simulink model "Lec_04_Storage10kWh"  (R2019b)
settings: Solver=VariableStepAuto  StartTime=0.0  StopTime=8400*3  MaxStep=0.05  RelTol=1e-3
undefined symbols (not defined in the file): Tcell0
libraries: simulink x5
settings Model: Creator=matm  LastModifiedBy=matm
settings SolverCC: ShapePreserveControl=EnableAll  SolverResetMethod=Robust
settings DataIOCC: ReturnWorkspaceOutputs=off
settings DebuggingCC: ArithmeticOperatorsInVariantConditions=warning
settings SFSimCC: SimUseLocalCustomCode=off  CustomCodeUndefinedFunction=UseInterfaceOnly
settings RTWCC: RTWUseLocalCustomCode=off
settings CodeAppCC: StateflowObjectComments=on

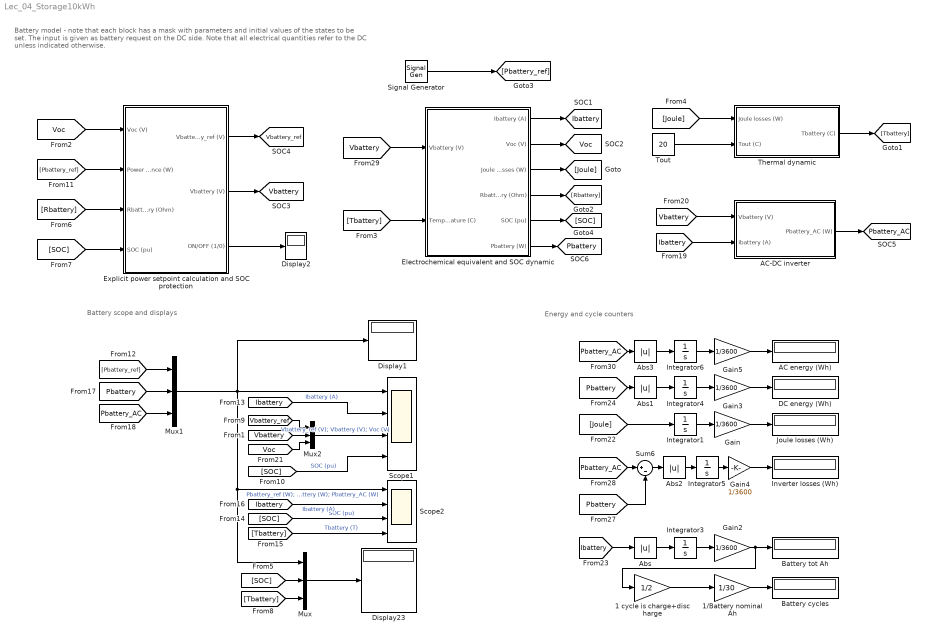
== system Lec_04_Storage10kWh ==
  note: Battery model - note that each block has a mask with parameters and initial values of the states to be set. The input is given as battery request on the DC side.
      | Note that all electrical quantities refer to the DC unless indicated otherwise.
  note: Battery scope and displays
  note: Energy and cycle counters
  1 cycle is charge+discharge : Gain  Gain=1/2
  1/Battery nominal Ah : Gain  Gain=1/30
  AC energy (Wh) : Display
  AC-DC inverter : Subsystem  mask{Inverter_Efficiency=0.95, Inverter_latency=0.1}
      mask prompts: Inverter_Efficiency "Inverter efficiency (pu)"; Inverter_latency "Inverter latency (s)"
  Abs{,1..3} (4 alike) : Abs
  Battery cycles : Display
  Battery tot Ah : Display
  DC energy (Wh) : Display
  Display1 : Display
  Display2 : Display
  Display23 : Display
  Electrochemical equivalent and SOC dynamic : Subsystem  mask{NumCellsSeries=100, NumCellsParallel=10, Ccell=3, SOC0=1}
      mask prompts: NumCellsSeries "Number of cells in Series"; NumCellsParallel "Number of cells in Parallel"; Ccell "Cell capacity (Ah)"; SOC0 "Initial state of charge (pu)"
  Explicit power setpoint calculation and SOC protection : Subsystem  mask{SOC_Max=1, SOC_Min=0, NumCellsSeries=100, CellVoltage_Max=4.2, CellVoltage_Min=2.6}
      mask prompts: SOC_Max "Max SOC (pu)"; SOC_Min "Min SOC (pu)"; NumCellsSeries "Number of celles in series"; CellVoltage_Max "Max cell voltage (V)"; CellVoltage_Min "Min cell voltage (V)"
      mask DialogControl DescTextVar Prompt: Power calculations and protections
  Gain{,2..5} (5 alike) : Gain  Gain=1/3600
  Integrator{1,3..6} (5 alike) : Integrator
  Inverter losses (Wh) : Display
  Joule losses (Wh) : Display
  Mux : Mux  Inputs=3
  Mux1 : Mux  Inputs=3
  Mux2 : Mux  Inputs=3
  Scope1 : Scope  NumInputPorts=4
  Scope2 : Scope  NumInputPorts=4
  Signal Generator : SignalGenerator  WaveForm=square  Amplitude=-10800  Frequency=1/(4200*2)
  Sum6 : Sum  Inputs=|+-
  Thermal dynamic : Subsystem  mask{Cth=72000, Rth=0.2}
      mask prompts: Cth "Thermal Capacitance (J/K)"; Rth "Thermal Resistance (K/W)"
      mask DialogControl DescTextVar Prompt: Thermal dynamic
  Tout : Constant  Value=20
  tag scope: Ibattery=global, Pbattery=global, Pbattery_AC=global, Vbattery=global, Vbattery_ref=global, Voc=global
  wires:
  [Vbattery] -> Electrochemical equivalent and SOC dynamic/1(Vbattery (V))
  Electrochemical equivalent and SOC dynamic/1(Ibattery (A)) -> [Ibattery]
  [Voc] -> Explicit power setpoint calculation and SOC protection/1(Voc (V))
  Electrochemical equivalent and SOC dynamic/2(Voc (V)) -> [Voc]
  Explicit power setpoint calculation and SOC protection/2(Vbattery (V)) -> [Vbattery]
  Electrochemical equivalent and SOC dynamic/3(Joule losses (W)) -> [Joule]
  Tout/1 -> Thermal dynamic/2(Tout (C))
  [Tbattery] -> Electrochemical equivalent and SOC dynamic/2(Temperature (C))
  Thermal dynamic/1(Tbattery (C)) -> [Tbattery]
  Mux/1 -> Display23/1
  Electrochemical equivalent and SOC dynamic/4(Rbattery (Ohm)) -> [Rbattery]
  [Rbattery] -> Explicit power setpoint calculation and SOC protection/3(Rbattery (Ohm))
  [SOC] -> Explicit power setpoint calculation and SOC protection/4(SOC (pu))
  Mux1/1 -> Display1/1, Scope1/1, Scope2/1, Mux/1  "Pbattery_ref (W); Pbattery (W); Pbattery_AC (W)"
  Explicit power setpoint calculation and SOC protection/3(ON/OFF (1/0)) -> Display2/1
  [Tbattery] -> Mux/3
  [Pbattery] -> Mux1/2
  [Pbattery_ref] -> Explicit power setpoint calculation and SOC protection/2(Power reference (W))
  [Pbattery_ref] -> Mux1/1
  [SOC] -> Scope1/4  "SOC (pu)"
  [Ibattery] -> Scope1/2  "Ibattery (A)"
  [SOC] -> Scope2/3  "SOC (pu)"
  [Tbattery] -> Scope2/4  "Tbattery (T)"
  [Ibattery] -> Scope2/2  "Ibattery (A)"
  Electrochemical equivalent and SOC dynamic/5(SOC (pu)) -> [SOC]
  Explicit power setpoint calculation and SOC protection/1(Vbattery_ref (V)) -> [Vbattery_ref]
  [Joule] -> Thermal dynamic/1(Joule losses (W))
  [Vbattery] -> AC-DC inverter/1(Vbattery (V))
  [Ibattery] -> AC-DC inverter/2(Ibattery (A))
  Electrochemical equivalent and SOC dynamic/6(Pbattery (W)) -> [Pbattery]
  [Pbattery_AC] -> Mux1/3
  [SOC] -> Mux/2
  AC-DC inverter/1(Pbattery_AC (W)) -> [Pbattery_AC]
  Mux2/1 -> Scope1/3  "Vbattery_ref (V); Vbattery (V); Voc (V)"
  [Vbattery] -> Mux2/2
  1/Battery nominal Ah/1 -> Battery cycles/1
  Integrator6/1 -> Gain5/1
  Gain2/1 -> 1 cycle is charge+discharge/1, Battery tot Ah/1
  [Pbattery_AC] -> Sum6/1
  Integrator5/1 -> Gain4/1
  [Pbattery_AC] -> Abs3/1
  Abs2/1 -> Integrator5/1
  Abs3/1 -> Integrator6/1
  Gain3/1 -> DC energy (Wh)/1
  Gain4/1 -> Inverter losses (Wh)/1
  Sum6/1 -> Abs2/1
  Integrator4/1 -> Gain3/1
  Abs1/1 -> Integrator4/1
  Integrator3/1 -> Gain2/1
  [Ibattery] -> Abs/1
  Gain/1 -> Joule losses (Wh)/1
  Integrator1/1 -> Gain/1
  Abs/1 -> Integrator3/1
  [Pbattery] -> Abs1/1
  [Joule] -> Integrator1/1
  [Pbattery] -> Sum6/2
  Gain5/1 -> AC energy (Wh)/1
  Signal Generator/1 -> [Pbattery_ref]
  [Vbattery_ref] -> Mux2/1
  [Voc] -> Mux2/3
  1 cycle is charge+discharge/1 -> 1/Battery nominal Ah/1

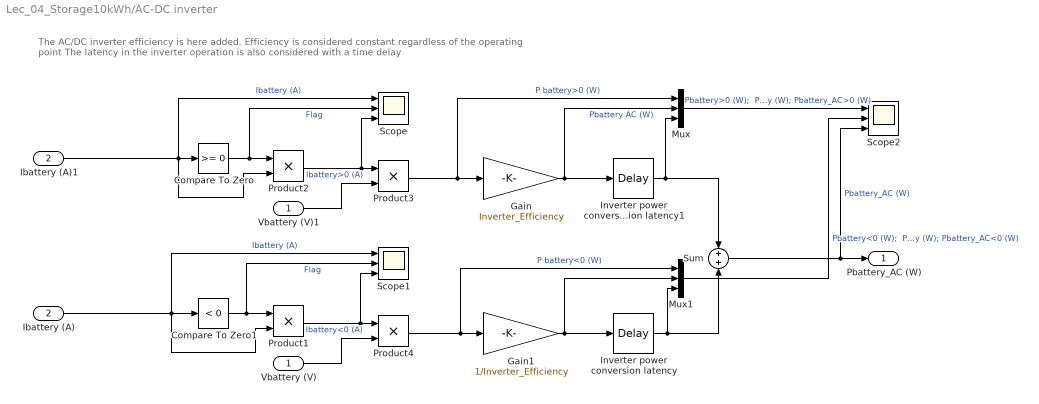
== system Lec_04_Storage10kWh/AC-DC inverter ==
  note: The AC/DC inverter efficiency is here added. Efficiency is considered constant regardless of the operating point
      | The latency in the inverter operation is also considered with a time delay
  Vbattery (V) : Inport
  Ibattery (A) : Inport  Port=2
  Compare To Zero : simulink/Logic and Bit Operations/Compare To Zero  relop=>=  OutDataTypeStr=boolean
  Compare To Zero1 : simulink/Logic and Bit Operations/Compare To Zero  relop=<  OutDataTypeStr=boolean
  Gain : Gain  Gain=Inverter_Efficiency
  Gain1 : Gain  Gain=1/Inverter_Efficiency
  Ibattery (A)1 : InportShadow  Port=2
  Inverter power conversion latency : TransportDelay  DelayTime=Inverter_latency
  Inverter power conversion latency1 : TransportDelay  DelayTime=Inverter_latency
  Mux : Mux  Inputs=3
  Mux1 : Mux  Inputs=3
  Product{1..4} (4 alike) : Product
  Scope : Scope  NumInputPorts=3
  Scope1 : Scope  NumInputPorts=3
  Scope2 : Scope  NumInputPorts=3
  Sum : Sum
  Vbattery (V)1 : InportShadow
  Pbattery_AC (W) : Outport
  wires:
  Sum/1 -> Scope2/3, Pbattery_AC (W)/1  "Pbattery_AC (W)"
  Ibattery (A)1/1 -> Scope/1, Product2/2, Compare To Zero/1  "Ibattery (A)"
  Compare To Zero/1 -> Scope/2, Product2/1  "Flag"
  Product2/1 -> Product3/1, Scope/3  "Ibattery>0 (A)"
  Product3/1 -> Mux/1, Gain/1  "P battery>0 (W)"
  Vbattery (V)1/1 -> Product3/2
  Vbattery (V)/1 -> Product4/2
  Product1/1 -> Scope1/3, Product4/1  "Ibattery<0 (A)"
  Compare To Zero1/1 -> Scope1/2, Product1/1  "Flag"
  Ibattery (A)/1 -> Scope1/1, Product1/2, Compare To Zero1/1  "Ibattery (A)"
  Product4/1 -> Mux1/1, Gain1/1  "P battery<0 (W)"
  Gain/1 -> Mux/2, Inverter power conversion latency1/1  "Pbattery AC (W)"
  Gain1/1 -> Mux1/2, Inverter power conversion latency/1
  Inverter power conversion latency1/1 -> Mux/3, Sum/1
  Inverter power conversion latency/1 -> Mux1/3, Sum/2
  Mux/1 -> Scope2/1  "Pbattery>0 (W);  Pbattery_AC>0 no delay (W); Pbattery_AC>0 (W)"
  Mux1/1 -> Scope2/2  "Pbattery<0 (W);  Pbattery_AC<0 no delay (W); Pbattery_AC<0 (W)"

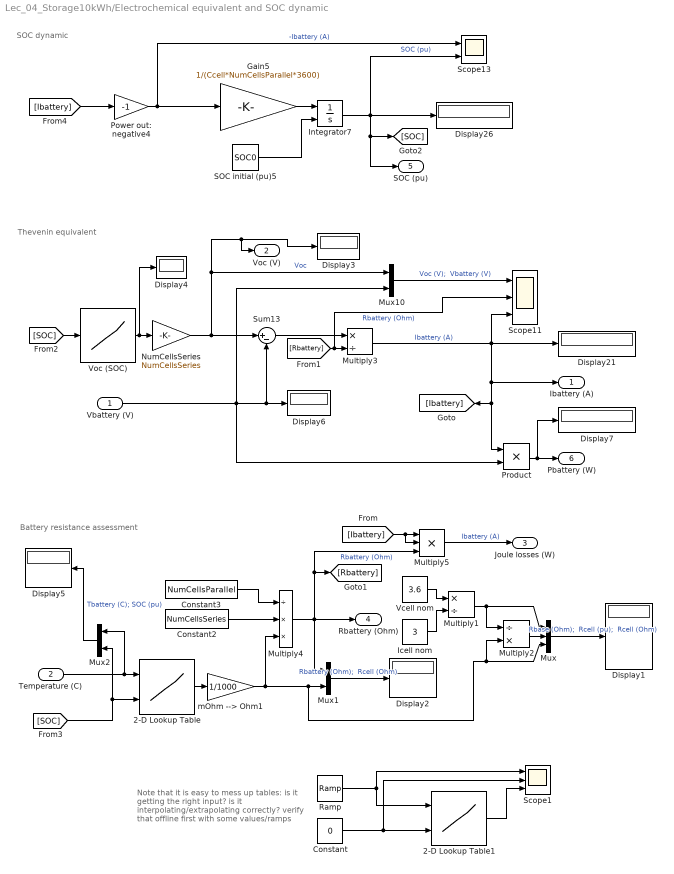
== system Lec_04_Storage10kWh/Electrochemical equivalent and SOC dynamic ==
  note: Note that it is easy to mess up tables: is it getting the right input? is it interpolating/extrapolating correctly? verify that offline first with some values/ramps
  note: SOC dynamic
  note: Battery resistance assessment
  note: Thevenin equivalent
  Vbattery (V) : Inport
  Temperature (C) : Inport  Port=2
  2-D Lookup Table : Lookup_n-D  BreakpointsForDimension1=[25 45]  BreakpointsForDimension2=[0 0.1 0.2 0.3 0.4 0.5 0.6 0.7 0.8 0.9 1]  Table=[54 36 33 33 32 32 31 33 33 34 41; 35 30 29 29 29 28 28 29 29 29 32]  ExtrapMethod=Clip  InternalRulePriority=Speed  RndMeth=Simplest  InputSameDT=on
  2-D Lookup Table1 : Lookup_n-D  BreakpointsForDimension1=[25 45]  BreakpointsForDimension2=[0 0.1 0.2 0.3 0.4 0.5 0.6 0.7 0.8 0.9 1]  Table=[54 36 33 33 32 32 31 33 33 34 41; 35 30 29 29 29 28 28 29 29 29 32]  ExtrapMethod=Clip  InternalRulePriority=Speed  RndMeth=Simplest  InputSameDT=on
  Constant : Constant  Value=0
  Constant2 : Constant  Value=NumCellsSeries
  Constant3 : Constant  Value=NumCellsParallel
  Display{1..7,21,26} (9 alike) : Display
  Gain5 : Gain  Gain=1/(Ccell*NumCellsParallel*3600)
  Icell nom : Constant  Value=3
  Integrator7 : Integrator  InitialConditionSource=external  InitialCondition=0.5  ZeroCross=off
  Multiply1 : Product  Inputs=*/
  Multiply2 : Product  Inputs=/*
  Multiply3 : Product  Inputs=*/
  Multiply4 : Product  Inputs=/**
  Multiply5 : Product  Inputs=***
  Mux : Mux  Inputs=3
  Mux1 : Mux  Inputs=2
  Mux10 : Mux  Inputs=2
  Mux2 : Mux  Inputs=2
  NumCellsSeries : Gain  Gain=NumCellsSeries
  Power out: negative4 : Gain  Gain=-1
  Product : Product
  Ramp : simulink/Sources/Ramp  slope=1  start=0  InitialOutput=0
  SOC initial (pu)5 : Constant  Value=SOC0
  Scope1 : Scope  NumInputPorts=3
  Scope11 : Scope  NumInputPorts=3
  Scope13 : Scope  NumInputPorts=2
  Sum13 : Sum  Inputs=|+-
  Vcell nom : Constant  Value=3.6
  Voc (SOC) : Lookup_n-D  NumberOfTableDimensions=1  BreakpointsForDimension1=[0 0.1 0.2 0.3 0.4 0.5 0.6 0.7 0.8 0.9 1]  Table=[2.85 3.19 3.39 3.52 3.65 3.73 3.82 3.92 4.01 4.07 4.19]  InternalRulePriority=Speed  RndMeth=Simplest  InputSameDT=on
  mOhm --> Ohm1 : Gain  Gain=1/1000
  Ibattery (A) : Outport  VectorParamsAs1DForOutWhenUnconnected=off
  Voc (V) : Outport  Port=2  VectorParamsAs1DForOutWhenUnconnected=off
  Joule losses (W) : Outport  Port=3  VectorParamsAs1DForOutWhenUnconnected=off
  Rbattery (Ohm) : Outport  Port=4  VectorParamsAs1DForOutWhenUnconnected=off
  SOC (pu) : Outport  Port=5  VectorParamsAs1DForOutWhenUnconnected=off
  Pbattery (W) : Outport  Port=6  VectorParamsAs1DForOutWhenUnconnected=off
  wires:
  Multiply3/1 -> Scope11/3, Display21/1, Product/1, [Ibattery], Ibattery (A)/1  "Ibattery (A)"
  [SOC] -> Voc (SOC)/1
  Mux10/1 -> Scope11/1  "Voc (V);  Vbattery (V)"
  Sum13/1 -> Multiply3/1
  Voc (SOC)/1 -> Display4/1, NumCellsSeries/1
  Vcell nom/1 -> Multiply1/1
  Icell nom/1 -> Multiply1/2
  2-D Lookup Table/1 -> mOhm --> Ohm1/1
  Multiply1/1 -> Mux/1, Multiply2/1
  Mux/1 -> Display1/1  "Rbase (Ohm);  Rcell (pu);  Rcell (Ohm)"
  Multiply2/1 -> Mux/2
  NumCellsSeries/1 -> Display3/1, Voc (V)/1, Mux10/1, Sum13/1  "Voc"
  Multiply5/1 -> Joule losses (W)/1  "Ibattery (A)"
  Mux1/1 -> Display2/1  "Rbattery (Ohm);  Rcell (Ohm)"
  Temperature (C)/1 -> Mux2/1, 2-D Lookup Table/1
  [SOC] -> Mux2/2, 2-D Lookup Table/2
  Multiply4/1 -> Rbattery (Ohm)/1, [Rbattery], Multiply5/3, Mux1/1  "Rbattery (Ohm)"
  mOhm --> Ohm1/1 -> Mux/3, Multiply2/2, Mux1/2, Multiply4/3
  Mux2/1 -> Display5/1  "Tbattery (C); SOC (pu)"
  Constant3/1 -> Multiply4/1
  Constant2/1 -> Multiply4/2
  Vbattery (V)/1 -> Product/2, Mux10/2, Display6/1, Sum13/2
  2-D Lookup Table1/1 -> Scope1/3
  Constant/1 -> Scope1/2, 2-D Lookup Table1/2
  Ramp/1 -> 2-D Lookup Table1/1, Scope1/1
  SOC initial (pu)5/1 -> Integrator7/2
  Gain5/1 -> Integrator7/1
  [Ibattery] -> Power out: negative4/1
  Integrator7/1 -> SOC (pu)/1, [SOC], Scope13/2, Display26/1  "SOC (pu)"
  Power out: negative4/1 -> Gain5/1, Scope13/1  "-Ibattery (A)"
  [Ibattery] -> Multiply5/2, Multiply5/1
  [Rbattery] -> Scope11/2, Multiply3/2  "Rbattery (Ohm)"
  Product/1 -> Display7/1, Pbattery (W)/1

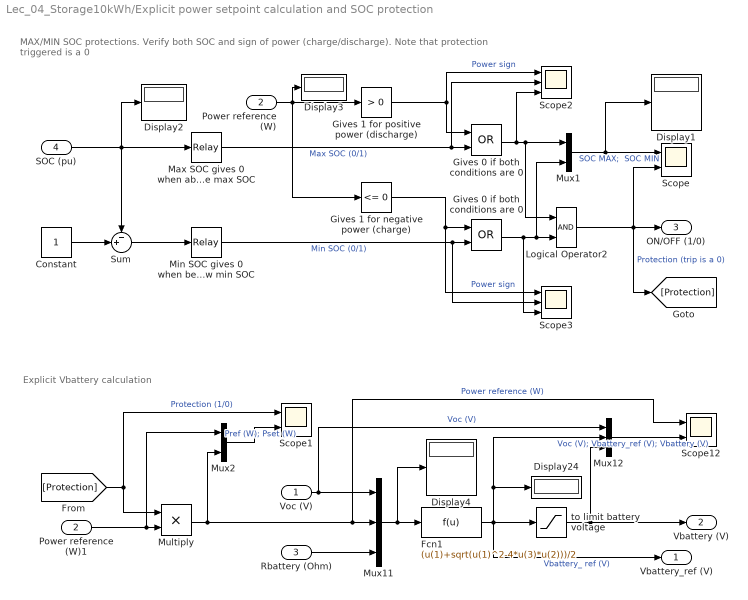
== system Lec_04_Storage10kWh/Explicit power setpoint calculation and SOC protection ==
  note: Explicit Vbattery calculation
  note: MAX/MIN SOC protections. Verify both SOC and sign of power (charge/discharge). Note that protection triggered is a 0
  Voc (V) : Inport
  Power reference (W) : Inport  Port=2
  Rbattery (Ohm) : Inport  Port=3
  SOC (pu) : Inport  Port=4
  Constant : Constant
  Display{1..4,24} (5 alike) : Display
  Fcn1 : Fcn  Expr=(u(1)+sqrt(u(1)^2-4*u(3)*u(2)))/2
  "Gives 0 if both conditions are 0 " : Logic  Operator=OR  AllPortsSameDT=off  OutDataTypeStr=boolean
  "Gives 0 if both conditions are 0 " : Logic  Operator=OR  AllPortsSameDT=off  OutDataTypeStr=boolean
  Gives 1 for negative power (charge) : simulink/Logic and Bit Operations/Compare To Zero  relop=<=  OutDataTypeStr=boolean
  Gives 1 for positive power (discharge) : simulink/Logic and Bit Operations/Compare To Zero  relop=>  OutDataTypeStr=boolean
  Logical Operator2 : Logic  AllPortsSameDT=off  OutDataTypeStr=boolean
  "Max SOC gives 0 when above max SOC " : Relay  OnSwitchValue=SOC_Max  OffSwitchValue=SOC_Max-0.01  OnOutputValue=0  OffOutputValue=1
  Min SOC gives 0 when below min SOC : Relay  OnSwitchValue=1-SOC_Min  OffSwitchValue=1-(SOC_Min+0.01)  OnOutputValue=0  OffOutputValue=1
  Multiply : Product
  Mux1 : Mux  Inputs=2
  Mux11 : Mux  Inputs=3
  Mux12 : Mux  Inputs=3
  Mux2 : Mux  Inputs=2
  Power reference (W)1 : InportShadow  Port=2
  Scope : Scope  NumInputPorts=2
  Scope1 : Scope  NumInputPorts=2
  Scope12 : Scope  NumInputPorts=2
  Scope2 : Scope  NumInputPorts=3
  Scope3 : Scope  NumInputPorts=3
  Sum : Sum  Inputs=-+|
  to limit battery voltage : Saturate  UpperLimit=CellVoltage_Max*NumCellsSeries  LowerLimit=CellVoltage_Min*NumCellsSeries
  Vbattery_ref (V) : Outport  VectorParamsAs1DForOutWhenUnconnected=off
  Vbattery (V) : Outport  Port=2  VectorParamsAs1DForOutWhenUnconnected=off
  ON/OFF (1/0) : Outport  Port=3  VectorParamsAs1DForOutWhenUnconnected=off
  wires:
  Voc (V)/1 -> Mux12/1, Mux11/1  "Voc (V)"
  Fcn1/1 -> Vbattery_ref (V)/1, Mux12/2, Display24/1, to limit battery voltage/1  "Vbattery_ ref (V)"
  Mux11/1 -> Display4/1, Fcn1/1
  Mux12/1 -> Scope12/2  "Voc (V); Vbattery_ref (V); Vbattery (V)"
  Constant/1 -> Sum/2
  SOC (pu)/1 -> Display2/1, Sum/1, "Max SOC gives 0 when above max SOC "/1
  Sum/1 -> Min SOC gives 0 when below min SOC/1
  Gives 1 for negative power (charge)/1 -> "Gives 0 if both conditions are 0 "/1, Scope3/1  "Power sign"
  Gives 1 for positive power (discharge)/1 -> "Gives 0 if both conditions are 0 "/1, Scope2/1  "Power sign"
  Power reference (W)/1 -> Gives 1 for positive power (discharge)/1, Gives 1 for negative power (charge)/1, Display3/1
  "Gives 0 if both conditions are 0 "/1 -> Mux1/1, Logical Operator2/1, Scope2/3
  "Gives 0 if both conditions are 0 "/1 -> Mux1/2, Logical Operator2/2, Scope3/3
  Logical Operator2/1 -> [Protection], ON/OFF (1/0)/1, Scope/2  "Protection (trip is a 0)"
  Mux1/1 -> Display1/1, Scope/1  "SOC MAX;  SOC MIN"
  Power reference (W)1/1 -> Mux2/1, Multiply/2
  [Protection] -> Scope1/1, Multiply/1  "Protection (1/0)"
  Multiply/1 -> Mux2/2, Scope12/1, Mux11/2  "Power reference (W)"
  Rbattery (Ohm)/1 -> Mux11/3
  Mux2/1 -> Scope1/2  "Pref (W); Pset (W)"
  Min SOC gives 0 when below min SOC/1 -> Scope3/2, "Gives 0 if both conditions are 0 "/2  "Min SOC (0/1)"
  to limit battery voltage/1 -> Vbattery (V)/1, Mux12/3
  "Max SOC gives 0 when above max SOC "/1 -> Scope2/2, "Gives 0 if both conditions are 0 "/2  "Max SOC (0/1)"

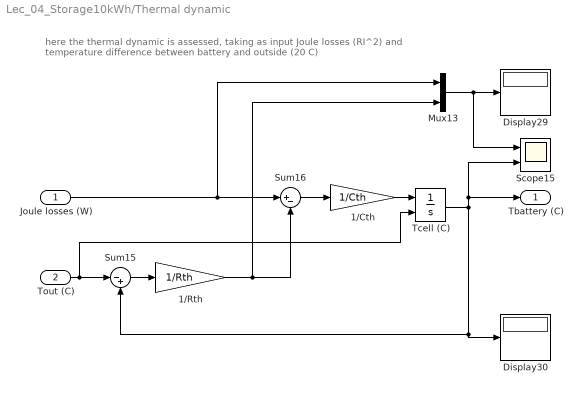
== system Lec_04_Storage10kWh/Thermal dynamic ==
  note: here the thermal dynamic is assessed, taking as input Joule losses (RI^2)
      | and temperature difference between battery and outside (20 C)
  Joule losses (W) : Inport
  Tout (C) : Inport  Port=2
  1/Cth : Gain  Gain=1/Cth
  1/Rth : Gain  Gain=1/Rth
  Display29 : Display
  Display30 : Display
  Mux13 : Mux  Inputs=2
  Scope15 : Scope  NumInputPorts=2
  Sum15 : Sum  Inputs=|-+
  Sum16 : Sum  Inputs=|+-
  Tcell (C) : Integrator  InitialConditionSource=external  InitialCondition=Tcell0  ZeroCross=off
  Tbattery (C) : Outport  VectorParamsAs1DForOutWhenUnconnected=off
  wires:
  1/Rth/1 -> Sum16/2, Mux13/2
  Joule losses (W)/1 -> Mux13/1, Sum16/1
  Sum16/1 -> 1/Cth/1
  Sum15/1 -> 1/Rth/1
  1/Cth/1 -> Tcell (C)/1
  Mux13/1 -> Display29/1, Scope15/1
  Tcell (C)/1 -> Tbattery (C)/1, Scope15/2, Display30/1, Sum15/2
  Tout (C)/1 -> Tcell (C)/2, Sum15/1
